simulink model "fpga_sim_disenio_filtro_iir"  (R2021b)
settings: Solver=VariableStepAuto  StartTime=0.0  StopTime=inf  RelTol=1e-3
InitFcn:
  | sim_disenio_filtro_iir_setting()
model workspace (MAT data in the model file):
  Fm = 100000
  a0 = 0.04539057
  a1 = 0
  a10 = 0
  a11 = 0
  a12 = 0
  a13 = 0
  a14 = 0
  a15 = 0
  a16 = 0
  a17 = 0
  a18 = 0
  a2 = 0
  a3 = 0
  a4 = 0
  a5 = 0
  a6 = 0
  a7 = 0
  a8 = 0
  a9 = 0
  b0 = 1
  b1 = 2.592371
  b10 = 0
  b11 = 0
  b12 = 0
  b13 = 0
  b14 = 0
  b15 = 0
  b16 = 0
  b17 = 0
  b18 = 0
  b2 = -2.84657
  b3 = 1.639055
  b4 = -0.491318
  b5 = 0.0609166
  b6 = 0
  b7 = 0
  b8 = 0
  b9 = 0
  z10_a = 12760
  z10_b = 12760
  z11_a = 12760
  z11_b = 12760
  z12_a = 12760
  z12_b = 12760
  z13_a = 12760
  z13_b = 12760
  z14_a = 12760
  z14_b = 12760
  z15_a = 12760
  z15_b = 12760
  z16_a = 12760
  z16_b = 12760
  z17_a = 12760
  z17_b = 12760
  z18_a = 12760
  z18_b = 12760
  z19_a = 12760
  z19_b = 12760
  z1_a = 12760
  z1_b = 12760
  z2_a = 100000
  z2_b = 100000
  z3_a = 100000
  z3_b = 100000
  z4_a = 100000
  z4_b = 100000
  z5_a = 100000
  z5_b = 100000
  z6_a = 100000
  z6_b = 100000
  z7_a = 100000
  z7_b = 100000
  z8_a = 100000
  z8_b = 100000
  z9_a = 100000
  z9_b = 100000
settings Model: Creator=fernando  LastModifiedBy=fernando
settings OptimizationCC: UseDivisionForNetSlopeComputation=on  UseFloatMulNetSlope=on  InheritOutputTypeSmallerThanSingle=on  DefaultUnderspecifiedDataType=single

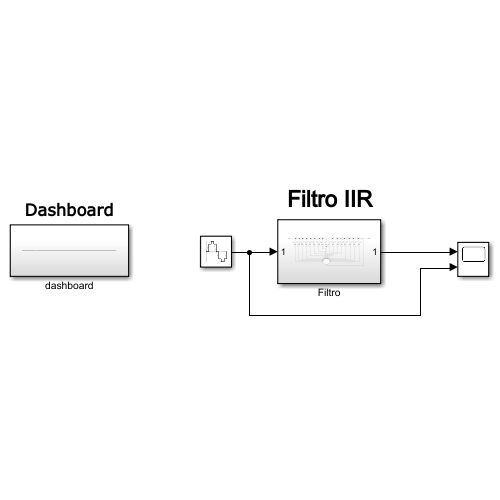
[thumbnail: Simulink's stored preview of the top-level diagram]
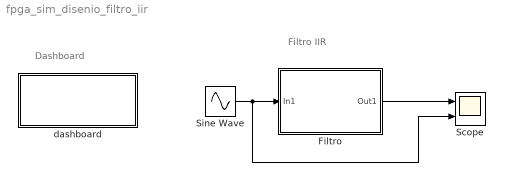
== system fpga_sim_disenio_filtro_iir ==
  note: Dashboard
  note: Filtro IIR
  Filtro : Subsystem
  Scope : Scope  NumInputPorts=2
  Sine Wave : Sin  Frequency=44003.62348676258  SampleTime=1/Fm
  dashboard : Subsystem
  wires:
  Filtro/1(Out1) -> Scope/1
  Sine Wave/1 -> Scope/2, Filtro/1(In1)

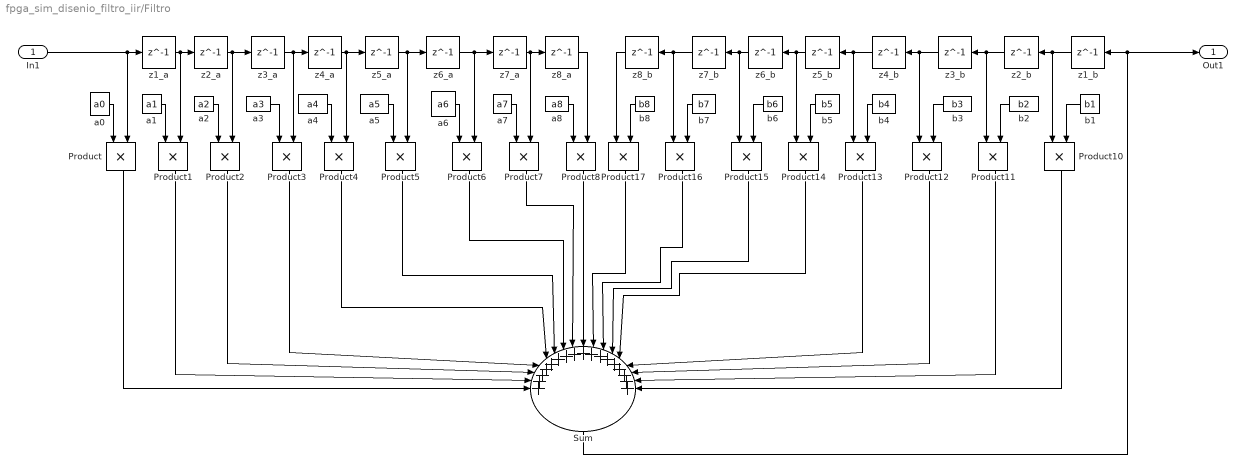
== system fpga_sim_disenio_filtro_iir/Filtro ==
  In1 : Inport
  Product{,1..8,10..17} (17 alike) : Product
  Sum : Sum  Inputs=+++++++++++++++++
  a0 : Constant  Value=a0  SampleTime=1/Fm
  a1 : Constant  Value=a1  SampleTime=1/Fm
  a2 : Constant  Value=a2  SampleTime=1/Fm
  a3 : Constant  Value=a3  SampleTime=1/Fm
  a4 : Constant  Value=a4  SampleTime=1/Fm
  a5 : Constant  Value=a5  SampleTime=1/Fm
  a6 : Constant  Value=a6  SampleTime=1/Fm
  a7 : Constant  Value=a7  SampleTime=1/Fm
  a8 : Constant  Value=a8  SampleTime=1/Fm
  b1 : Constant  Value=b1  SampleTime=1/Fm
  b2 : Constant  Value=b2  SampleTime=1/Fm
  b3 : Constant  Value=b3  SampleTime=1/Fm
  b4 : Constant  Value=b4  SampleTime=1/Fm
  b5 : Constant  Value=b5  SampleTime=1/Fm
  b6 : Constant  Value=b6  SampleTime=1/Fm
  b7 : Constant  Value=b7  SampleTime=1/Fm
  b8 : Constant  Value=b8  SampleTime=1/Fm
  z1_a : Delay  DelayLength=1  InitialCondition=0  SampleTime=1/Fm
  z1_b : Delay  DelayLength=1  InitialCondition=0  SampleTime=1/Fm
  z2_a : Delay  DelayLength=1  InitialCondition=0  SampleTime=1/Fm
  z2_b : Delay  DelayLength=1  InitialCondition=0  SampleTime=1/Fm
  z3_a : Delay  DelayLength=1  InitialCondition=0  SampleTime=1/Fm
  z3_b : Delay  DelayLength=1  InitialCondition=0  SampleTime=1/Fm
  z4_a : Delay  DelayLength=1  InitialCondition=0  SampleTime=1/Fm
  z4_b : Delay  DelayLength=1  InitialCondition=0  SampleTime=1/Fm
  z5_a : Delay  DelayLength=1  InitialCondition=0  SampleTime=1/Fm
  z5_b : Delay  DelayLength=1  InitialCondition=0  SampleTime=1/Fm
  z6_a : Delay  DelayLength=1  InitialCondition=0  SampleTime=1/Fm
  z6_b : Delay  DelayLength=1  InitialCondition=0  SampleTime=1/Fm
  z7_a : Delay  DelayLength=1  InitialCondition=0  SampleTime=1/Fm
  z7_b : Delay  DelayLength=1  InitialCondition=0  SampleTime=1/Fm
  z8_a : Delay  DelayLength=1  InitialCondition=0  SampleTime=1/Fm
  z8_b : Delay  DelayLength=1  InitialCondition=0  SampleTime=1/Fm
  Out1 : Outport
  wires:
  z1_a/1 -> z2_a/1, Product1/2
  a0/1 -> Product/1
  a4/1 -> Product4/1
  Product12/1 -> Sum/15
  Product11/1 -> Sum/16
  Product3/1 -> Sum/4
  z4_b/1 -> Product13/2, z5_b/1
  z7_a/1 -> z8_a/1, Product7/2
  z7_b/1 -> z8_b/1, Product16/2
  a1/1 -> Product1/1
  z8_a/1 -> Product8/2
  Product10/1 -> Sum/17
  b2/1 -> Product11/1
  z2_a/1 -> z3_a/1, Product2/2
  b5/1 -> Product14/1
  a6/1 -> Product6/1
  Product6/1 -> Sum/7
  a5/1 -> Product5/1
  a3/1 -> Product3/1
  Product16/1 -> Sum/11
  z6_b/1 -> Product15/2, z7_b/1
  Product2/1 -> Sum/3
  a7/1 -> Product7/1
  z6_a/1 -> z7_a/1, Product6/2
  Product14/1 -> Sum/13
  Product/1 -> Sum/1
  z5_a/1 -> z6_a/1, Product5/2
  Product4/1 -> Sum/5
  In1/1 -> z1_a/1, Product/2
  z3_a/1 -> z4_a/1, Product3/2
  z1_b/1 -> Product10/2, z2_b/1
  a2/1 -> Product2/1
  z4_a/1 -> z5_a/1, Product4/2
  z5_b/1 -> z6_b/1, Product14/2
  b3/1 -> Product12/1
  Product1/1 -> Sum/2
  Sum/1 -> z1_b/1, Out1/1
  b7/1 -> Product16/1
  b1/1 -> Product10/1
  z8_b/1 -> Product17/2
  z2_b/1 -> Product11/2, z3_b/1
  Product7/1 -> Sum/8
  Product17/1 -> Sum/10
  a8/1 -> Product8/1
  b4/1 -> Product13/1
  Product15/1 -> Sum/12
  Product5/1 -> Sum/6
  b8/1 -> Product17/1
  Product13/1 -> Sum/14
  Product8/1 -> Sum/9
  z3_b/1 -> z4_b/1, Product12/2
  b6/1 -> Product15/1

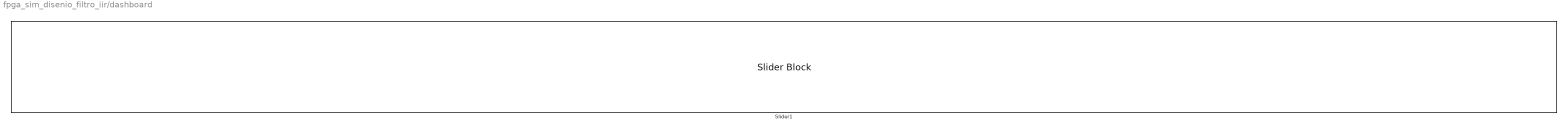
== system fpga_sim_disenio_filtro_iir/dashboard ==
  Slider1 : SliderBlock  ScaleMin=1  ScaleMax=314159.26535897929  TickInterval=6283.1853071795858
